simulink model "case3"  (R2024b)
settings: Solver=FixedStepAuto  StartTime=0  StopTime=1  FixedStep=1e-7  RelTol=1e-3
values from neighbouring files (symbols this model uses):
  SG_D_1_D = 0.01056    [IEEE9_case_parameters.m]    (also in case1_parameters.m; case2_parameters.m; case3_parameters.m; case4_parameters.m)
  SG_D_1_EnableSaturation = 0    [IEEE9_case_parameters.m]    (also in case1_parameters.m; case2_parameters.m; case3_parameters.m; case4_parameters.m)
  SG_D_1_f0 = 60    [IEEE9_case_parameters.m]    (also in case1_parameters.m; case2_parameters.m; case3_parameters.m; case4_parameters.m)
  SG_D_1_H = 7.5    [IEEE9_case_parameters.m]    (also in case1_parameters.m; case2_parameters.m; case3_parameters.m; case4_parameters.m)
  SG_D_1_K_A = 20    [IEEE9_case_parameters.m]    (also in case1_parameters.m; case2_parameters.m; case3_parameters.m; case4_parameters.m)
  SG_D_1_K_E = 1.000000e+1    (= 10)    [IEEE9_case_parameters.m]    (also in case1_parameters.m; case2_parameters.m; case3_parameters.m; case4_parameters.m)
  SG_D_1_K_F = 2.363    [IEEE9_case_parameters.m]    (also in case1_parameters.m; case2_parameters.m; case3_parameters.m; case4_parameters.m)
  SG_D_1_K_s = 0.5    [IEEE9_case_parameters.m]    (also in case1_parameters.m = 5; case2_parameters.m = 5; case3_parameters.m = 5; case4_parameters.m = 5)
  SG_D_1_R_a = 0.001088    [IEEE9_case_parameters.m]    (also in case1_parameters.m; case2_parameters.m; case3_parameters.m; case4_parameters.m)
  SG_D_1_S_A = 1    [IEEE9_case_parameters.m]    (also in case1_parameters.m; case2_parameters.m; case3_parameters.m; case4_parameters.m)
  SG_D_1_S_B = 0.103    [IEEE9_case_parameters.m]    (also in case1_parameters.m; case2_parameters.m; case3_parameters.m; case4_parameters.m)
  SG_D_1_S_N = 10.659857    [IEEE9_case_parameters.m]    (also in case1_parameters.m; case2_parameters.m; case3_parameters.m; case4_parameters.m)
  SG_D_1_SpeedPara = 200    [IEEE9_case_parameters.m]    (also in case1_parameters.m; case2_parameters.m; case3_parameters.m; case4_parameters.m)
  SG_D_1_T_0 = 0.720173    [IEEE9_case_parameters.m]    (also in case1_parameters.m = 0.755522; case2_parameters.m = 0.808931; case3_parameters.m = 0.869402; case4_parameters.m = 0.729316)
  SG_D_1_T_1 = 0.3    [IEEE9_case_parameters.m]    (also in case1_parameters.m; case2_parameters.m; case3_parameters.m; case4_parameters.m)
  SG_D_1_T_2 = 0.05    [IEEE9_case_parameters.m]    (also in case1_parameters.m; case2_parameters.m; case3_parameters.m; case4_parameters.m)
  SG_D_1_T_3 = 0.02    [IEEE9_case_parameters.m]    (also in case1_parameters.m; case2_parameters.m; case3_parameters.m; case4_parameters.m)
  SG_D_1_T_4 = 0.005    [IEEE9_case_parameters.m]    (also in case1_parameters.m; case2_parameters.m; case3_parameters.m; case4_parameters.m)
  SG_D_1_T_A = 0.02    [IEEE9_case_parameters.m]    (also in case1_parameters.m; case2_parameters.m; case3_parameters.m; case4_parameters.m)
  SG_D_1_T_dd = 8.000000e+0    (= 8)    [IEEE9_case_parameters.m]    (also in case1_parameters.m; case2_parameters.m; case3_parameters.m; case4_parameters.m)
  SG_D_1_T_ddd = 0.04    [IEEE9_case_parameters.m]    (also in case1_parameters.m; case2_parameters.m; case3_parameters.m; case4_parameters.m)
  SG_D_1_T_E = 0.314    [IEEE9_case_parameters.m]    (also in case1_parameters.m; case2_parameters.m; case3_parameters.m; case4_parameters.m)
  SG_D_1_T_F = 0.35    [IEEE9_case_parameters.m]    (also in case1_parameters.m; case2_parameters.m; case3_parameters.m; case4_parameters.m)
  SG_D_1_T_qd = 0.8    [IEEE9_case_parameters.m]    (also in case1_parameters.m; case2_parameters.m; case3_parameters.m; case4_parameters.m)
  SG_D_1_T_qdd = 0.02    [IEEE9_case_parameters.m]    (also in case1_parameters.m; case2_parameters.m; case3_parameters.m; case4_parameters.m)
  SG_D_1_T_speed = 0.1    [IEEE9_case_parameters.m]    (also in case1_parameters.m = 200; case2_parameters.m = 200; case3_parameters.m = 200; case4_parameters.m = 200)
  SG_D_1_T_w = 0.5    [IEEE9_case_parameters.m]    (also in case1_parameters.m; case2_parameters.m; case3_parameters.m; case4_parameters.m)
  SG_D_1_V_ref = 1.990276    [IEEE9_case_parameters.m]    (also in case1_parameters.m = 2.042296; case2_parameters.m = 2.051388; case3_parameters.m = 2.089584; case4_parameters.m = 2.01845)
  SG_D_1_w_ref = 376.991118    [IEEE9_case_parameters.m]    (also in case1_parameters.m; case2_parameters.m; case3_parameters.m; case4_parameters.m)
  SG_D_1_wb = 6.000000e+1    (= 60)    [IEEE9_case_parameters.m]    (also in case1_parameters.m; case2_parameters.m; case3_parameters.m; case4_parameters.m)
  SG_D_1_x_d = 1.9    [IEEE9_case_parameters.m]    (also in case1_parameters.m; case2_parameters.m; case3_parameters.m; case4_parameters.m)
  SG_D_1_x_dd = 0.302    [IEEE9_case_parameters.m]    (also in case1_parameters.m; case2_parameters.m; case3_parameters.m; case4_parameters.m)
  SG_D_1_x_ddd = 0.204    [IEEE9_case_parameters.m]    (also in case1_parameters.m; case2_parameters.m; case3_parameters.m; case4_parameters.m)
  SG_D_1_x_l = 0.05    [IEEE9_case_parameters.m]    (also in case1_parameters.m; case2_parameters.m; case3_parameters.m; case4_parameters.m)
  SG_D_1_x_q = 1.3    [IEEE9_case_parameters.m]    (also in case1_parameters.m; case2_parameters.m; case3_parameters.m; case4_parameters.m)
  SG_D_1_x_qd = 0.5    [IEEE9_case_parameters.m]    (also in case1_parameters.m; case2_parameters.m; case3_parameters.m; case4_parameters.m)
  SG_D_1_x_qdd = 0.3    [IEEE9_case_parameters.m]    (also in case1_parameters.m; case2_parameters.m; case3_parameters.m; case4_parameters.m)
  SG_D_2_D = 0.02    [IEEE9_case_parameters.m]    (also in case1_parameters.m; case2_parameters.m; case3_parameters.m; case4_parameters.m)
  SG_D_2_EnableSaturation = 0    [IEEE9_case_parameters.m]    (also in case1_parameters.m; case2_parameters.m; case3_parameters.m; case4_parameters.m)
  SG_D_2_f0 = 60    [IEEE9_case_parameters.m]    (also in case1_parameters.m; case2_parameters.m; case3_parameters.m; case4_parameters.m)
  SG_D_2_H = 8.000000e+0    (= 8)    [IEEE9_case_parameters.m]    (also in case1_parameters.m; case2_parameters.m; case3_parameters.m; case4_parameters.m)
  SG_D_2_K_A = 20    [IEEE9_case_parameters.m]    (also in case1_parameters.m; case2_parameters.m; case3_parameters.m; case4_parameters.m)
  SG_D_2_K_E = 1.000000e+1    (= 10)    [IEEE9_case_parameters.m]    (also in case1_parameters.m; case2_parameters.m; case3_parameters.m; case4_parameters.m)
  SG_D_2_K_F = 2.363    [IEEE9_case_parameters.m]    (also in case1_parameters.m; case2_parameters.m; case3_parameters.m; case4_parameters.m)
  SG_D_2_K_s = 0.5    [IEEE9_case_parameters.m]    (also in case1_parameters.m = 4; case2_parameters.m = 4; case3_parameters.m = 4; case4_parameters.m = 4)
  SG_D_2_R_a = 0.001088    [IEEE9_case_parameters.m]    (also in case1_parameters.m; case2_parameters.m; case3_parameters.m; case4_parameters.m)
  SG_D_2_S_A = 1    [IEEE9_case_parameters.m]    (also in case1_parameters.m; case2_parameters.m; case3_parameters.m; case4_parameters.m)
  SG_D_2_S_B = 0.103    [IEEE9_case_parameters.m]    (also in case1_parameters.m; case2_parameters.m; case3_parameters.m; case4_parameters.m)
  SG_D_2_S_N = 10.659857    [IEEE9_case_parameters.m]    (also in case1_parameters.m; case2_parameters.m; case3_parameters.m; case4_parameters.m)
  SG_D_2_SpeedPara = 200    [IEEE9_case_parameters.m]    (also in case1_parameters.m; case2_parameters.m; case3_parameters.m; case4_parameters.m)
  SG_D_2_T_0 = 1.632913    [IEEE9_case_parameters.m]    (also in case1_parameters.m = 1.632925; case2_parameters.m = 1.632915; case3_parameters.m = 1.632914; case4_parameters.m = 1.632927)
  SG_D_2_T_1 = 0.2    [IEEE9_case_parameters.m]    (also in case1_parameters.m; case2_parameters.m; case3_parameters.m; case4_parameters.m)
  SG_D_2_T_2 = 0.05    [IEEE9_case_parameters.m]    (also in case1_parameters.m; case2_parameters.m; case3_parameters.m; case4_parameters.m)
  SG_D_2_T_3 = 0.02    [IEEE9_case_parameters.m]    (also in case1_parameters.m; case2_parameters.m; case3_parameters.m; case4_parameters.m)
  SG_D_2_T_4 = 0.005    [IEEE9_case_parameters.m]    (also in case1_parameters.m; case2_parameters.m; case3_parameters.m; case4_parameters.m)
  SG_D_2_T_A = 0.02    [IEEE9_case_parameters.m]    (also in case1_parameters.m; case2_parameters.m; case3_parameters.m; case4_parameters.m)
  SG_D_2_T_dd = 7.9    [IEEE9_case_parameters.m]    (also in case1_parameters.m; case2_parameters.m; case3_parameters.m; case4_parameters.m)
  SG_D_2_T_ddd = 0.04    [IEEE9_case_parameters.m]    (also in case1_parameters.m; case2_parameters.m; case3_parameters.m; case4_parameters.m)
  SG_D_2_T_E = 0.314    [IEEE9_case_parameters.m]    (also in case1_parameters.m; case2_parameters.m; case3_parameters.m; case4_parameters.m)
  SG_D_2_T_F = 0.35    [IEEE9_case_parameters.m]    (also in case1_parameters.m; case2_parameters.m; case3_parameters.m; case4_parameters.m)
  SG_D_2_T_qd = 0.8    [IEEE9_case_parameters.m]    (also in case1_parameters.m; case2_parameters.m; case3_parameters.m; case4_parameters.m)
  SG_D_2_T_qdd = 0.015    [IEEE9_case_parameters.m]    (also in case1_parameters.m; case2_parameters.m; case3_parameters.m; case4_parameters.m)
  SG_D_2_T_speed = 0.1    [IEEE9_case_parameters.m]    (also in case1_parameters.m = 150; case2_parameters.m = 150; case3_parameters.m = 150; case4_parameters.m = 150)
  SG_D_2_T_w = 0.35    [IEEE9_case_parameters.m]    (also in case1_parameters.m; case2_parameters.m; case3_parameters.m; case4_parameters.m)
  SG_D_2_V_ref = 2.58547    [IEEE9_case_parameters.m]    (also in case1_parameters.m = 2.597896; case2_parameters.m = 2.587136; case3_parameters.m = 2.586042; case4_parameters.m = 2.599679)
  SG_D_2_w_ref = 376.991118    [IEEE9_case_parameters.m]    (also in case1_parameters.m; case2_parameters.m; case3_parameters.m; case4_parameters.m)
  SG_D_2_wb = 6.000000e+1    (= 60)    [IEEE9_case_parameters.m]    (also in case1_parameters.m; case2_parameters.m; case3_parameters.m; case4_parameters.m)
  SG_D_2_x_d = 1.8    [IEEE9_case_parameters.m]    (also in case1_parameters.m; case2_parameters.m; case3_parameters.m; case4_parameters.m)
  SG_D_2_x_dd = 0.302    [IEEE9_case_parameters.m]    (also in case1_parameters.m; case2_parameters.m; case3_parameters.m; case4_parameters.m)
  SG_D_2_x_ddd = 0.204    [IEEE9_case_parameters.m]    (also in case1_parameters.m; case2_parameters.m; case3_parameters.m; case4_parameters.m)
  SG_D_2_x_l = 0.05    [IEEE9_case_parameters.m]    (also in case1_parameters.m; case2_parameters.m; case3_parameters.m; case4_parameters.m)
  SG_D_2_x_q = 1.25    [IEEE9_case_parameters.m]    (also in case1_parameters.m; case2_parameters.m; case3_parameters.m; case4_parameters.m)
  SG_D_2_x_qd = 0.5    [IEEE9_case_parameters.m]    (also in case1_parameters.m; case2_parameters.m; case3_parameters.m; case4_parameters.m)
  SG_D_2_x_qdd = 0.3    [IEEE9_case_parameters.m]    (also in case1_parameters.m; case2_parameters.m; case3_parameters.m; case4_parameters.m)
  SG_D_3_D = 0.02    [IEEE9_case_parameters.m]    (also in case1_parameters.m; case2_parameters.m; case3_parameters.m; case4_parameters.m)
  SG_D_3_EnableSaturation = 0    [IEEE9_case_parameters.m]    (also in case1_parameters.m; case2_parameters.m; case3_parameters.m; case4_parameters.m)
  SG_D_3_f0 = 60    [IEEE9_case_parameters.m]    (also in case1_parameters.m; case2_parameters.m; case3_parameters.m; case4_parameters.m)
  SG_D_3_H = 7.7    [IEEE9_case_parameters.m]    (also in case1_parameters.m; case2_parameters.m; case3_parameters.m; case4_parameters.m)
  SG_D_3_K_A = 20    [IEEE9_case_parameters.m]    (also in case1_parameters.m; case2_parameters.m; case3_parameters.m; case4_parameters.m)
  SG_D_3_K_E = 1.000000e+1    (= 10)    [IEEE9_case_parameters.m]    (also in case1_parameters.m; case2_parameters.m; case3_parameters.m; case4_parameters.m)
  SG_D_3_K_F = 2.363    [IEEE9_case_parameters.m]    (also in case1_parameters.m; case2_parameters.m; case3_parameters.m; case4_parameters.m)
  SG_D_3_K_s = 0.2    [IEEE9_case_parameters.m]    (also in case1_parameters.m = 2; case2_parameters.m = 2; case3_parameters.m = 2; case4_parameters.m = 2)
  SG_D_3_R_a = 0.001088    [IEEE9_case_parameters.m]    (also in case1_parameters.m; case2_parameters.m; case3_parameters.m; case4_parameters.m)
  SG_D_3_S_A = 1    [IEEE9_case_parameters.m]    (also in case1_parameters.m; case2_parameters.m; case3_parameters.m; case4_parameters.m)
  SG_D_3_S_B = 0.103    [IEEE9_case_parameters.m]    (also in case1_parameters.m; case2_parameters.m; case3_parameters.m; case4_parameters.m)
  SG_D_3_S_N = 10.659857    [IEEE9_case_parameters.m]    (also in case1_parameters.m; case2_parameters.m; case3_parameters.m; case4_parameters.m)
  SG_D_3_SpeedPara = 200    [IEEE9_case_parameters.m]    (also in case1_parameters.m; case2_parameters.m; case3_parameters.m; case4_parameters.m)
  SG_D_3_T_0 = 0.850788    [IEEE9_case_parameters.m]    (also in case1_parameters.m = 0.850786; case2_parameters.m = 0.850787; case3_parameters.m; case4_parameters.m = 0.850786)
  SG_D_3_T_1 = 0.2    [IEEE9_case_parameters.m]    (also in case1_parameters.m; case2_parameters.m; case3_parameters.m; case4_parameters.m)
  SG_D_3_T_2 = 0.05    [IEEE9_case_parameters.m]    (also in case1_parameters.m; case2_parameters.m; case3_parameters.m; case4_parameters.m)
  SG_D_3_T_3 = 0.02    [IEEE9_case_parameters.m]    (also in case1_parameters.m; case2_parameters.m; case3_parameters.m; case4_parameters.m)
  SG_D_3_T_4 = 0.005    [IEEE9_case_parameters.m]    (also in case1_parameters.m; case2_parameters.m; case3_parameters.m; case4_parameters.m)
  SG_D_3_T_A = 0.02    [IEEE9_case_parameters.m]    (also in case1_parameters.m; case2_parameters.m; case3_parameters.m; case4_parameters.m)
  SG_D_3_T_dd = 8.1    [IEEE9_case_parameters.m]    (also in case1_parameters.m; case2_parameters.m; case3_parameters.m; case4_parameters.m)
  SG_D_3_T_ddd = 0.04    [IEEE9_case_parameters.m]    (also in case1_parameters.m; case2_parameters.m; case3_parameters.m; case4_parameters.m)
  SG_D_3_T_E = 0.314    [IEEE9_case_parameters.m]    (also in case1_parameters.m; case2_parameters.m; case3_parameters.m; case4_parameters.m)
  SG_D_3_T_F = 0.35    [IEEE9_case_parameters.m]    (also in case1_parameters.m; case2_parameters.m; case3_parameters.m; case4_parameters.m)
  SG_D_3_T_qd = 0.8    [IEEE9_case_parameters.m]    (also in case1_parameters.m; case2_parameters.m; case3_parameters.m; case4_parameters.m)
  SG_D_3_T_qdd = 0.015    [IEEE9_case_parameters.m]    (also in case1_parameters.m; case2_parameters.m; case3_parameters.m; case4_parameters.m)
  SG_D_3_T_speed = 0.1    [IEEE9_case_parameters.m]    (also in case1_parameters.m = 180; case2_parameters.m = 180; case3_parameters.m = 180; case4_parameters.m = 180)
  SG_D_3_T_w = 0.4    [IEEE9_case_parameters.m]    (also in case1_parameters.m; case2_parameters.m; case3_parameters.m; case4_parameters.m)
  SG_D_3_V_ref = 1.892727    [IEEE9_case_parameters.m]    (also in case1_parameters.m = 1.906439; case2_parameters.m = 1.895535; case3_parameters.m = 1.892105; case4_parameters.m = 1.906598)
  SG_D_3_w_ref = 376.991118    [IEEE9_case_parameters.m]    (also in case1_parameters.m; case2_parameters.m; case3_parameters.m; case4_parameters.m)
  SG_D_3_wb = 6.000000e+1    (= 60)    [IEEE9_case_parameters.m]    (also in case1_parameters.m; case2_parameters.m; case3_parameters.m; case4_parameters.m)
  SG_D_3_x_d = 1.85    [IEEE9_case_parameters.m]    (also in case1_parameters.m; case2_parameters.m; case3_parameters.m; case4_parameters.m)
  SG_D_3_x_dd = 0.302    [IEEE9_case_parameters.m]    (also in case1_parameters.m; case2_parameters.m; case3_parameters.m; case4_parameters.m)
  SG_D_3_x_ddd = 0.204    [IEEE9_case_parameters.m]    (also in case1_parameters.m; case2_parameters.m; case3_parameters.m; case4_parameters.m)
  SG_D_3_x_l = 0.05    [IEEE9_case_parameters.m]    (also in case1_parameters.m; case2_parameters.m; case3_parameters.m; case4_parameters.m)
  SG_D_3_x_q = 1.2    [IEEE9_case_parameters.m]    (also in case1_parameters.m; case2_parameters.m; case3_parameters.m; case4_parameters.m)
  SG_D_3_x_qd = 0.5    [IEEE9_case_parameters.m]    (also in case1_parameters.m; case2_parameters.m; case3_parameters.m; case4_parameters.m)
  SG_D_3_x_qdd = 0.3    [IEEE9_case_parameters.m]    (also in case1_parameters.m; case2_parameters.m; case3_parameters.m; case4_parameters.m)
(part 8 of 12)

== system case3/SG_D_2/d_psi_d_SG_D_2_block ==
  note: d_psi_d_SG_D_2 in case3
      | $2\,\pi \,f_{0}\,\left(v_{d,\mathrm{SG},D,2}\,\sin\left(\theta _{\mathrm{SG},D,2}\right)-v_{q,\mathrm{SG},D,2}\,\cos\left(\theta _{\mathrm{SG},D,2}\right)+\frac{R_{a}\,\left(\frac{\psi _{\mathrm{1d},\mathrm{SG},D,2}\,\left(x_{\mathrm{dd}}-x_{\mathrm{ddd}}\right)}{x_{\mathrm{dd}}-x_{l}}-\psi _{d,\mathrm{SG},D,2}+\frac{\psi _{\mathrm{fd},\mathrm{SG},D,2}\,\left(x_{\mathrm{ddd}}-x_{l}\right)}{x_{\mathrm{dd}}-x_{l}}\right)}{x_{\mathrm{ddd}}}+\frac{\psi _{q,\mathrm{SG},D,2}\,w_{\mathrm{SG},D,2}}{2\,f_{0}\,\pi }\right)$
      | Automatically generated on 2025-10-31 18:59:51 .
  State_psi_1d_SG_D_2_d85f5 : Inport
  State_psi_d_SG_D_2_2712a : Inport  Port=2
  State_psi_fd_SG_D_2_3f7c9 : Inport  Port=3
  Input_v_d_SG_D_2_8a747 : Inport  Port=4
  State_theta_SG_D_2_fc879 : Inport  Port=5
  Input_v_q_SG_D_2_bd396 : Inport  Port=6
  State_theta_SG_D_2_1886b : Inport  Port=7
  State_psi_q_SG_D_2_f5763 : Inport  Port=8
  State_w_SG_D_2_5f49e : Inport  Port=9
  Add_4c6a2 : Sum
  Add_a24d9 : Sum
  Constant_-1_feb9b : Constant  Value=-1
  Constant_-2.0_5ab6a : Constant  Value=-2.0
  Constant_2.0_914c1 : Constant  Value=2.0
  Constant_R_a_7ff2e : Constant  Value=R_a
  Constant_f0_1428f : Constant  Value=f0
  Constant_f0_1bd3e : Constant  Value=f0
  Constant_pi_05147 : Constant  Value=pi
  Constant_pi_d2189 : Constant  Value=pi
  Constant_x_dd_3b685 : Constant  Value=x_dd
  Constant_x_dd_d1044 : Constant  Value=x_dd
  Constant_x_dd_fa650 : Constant  Value=x_dd
  Constant_x_ddd_117c4 : Constant  Value=x_ddd
  Constant_x_ddd_cc768 : Constant  Value=x_ddd
  Constant_x_ddd_feb60 : Constant  Value=x_ddd
  Constant_x_l_14631 : Constant  Value=x_l
  Constant_x_l_2aec7 : Constant  Value=x_l
  Constant_x_l_a18c8 : Constant  Value=x_l
  Divide_3d9c5 : Product  Inputs=*/
  Divide_6089c : Product  Inputs=*/
  Divide_65062 : Product  Inputs=*/
  Divide_be36f : Product  Inputs=*/
  MathFunc_cos_04d6f : Trigonometry  Operator=cos
  MathFunc_sin_14dfb : Trigonometry
  Product_01511 : Product
  Product_10db0 : Product
  Product_37ec0 : Product
  Product_3b24f : Product
  Product_8fc40 : Product
  Product_9439a : Product
  Product_a26ec : Product
  Product_ac62c : Product
  Product_c5a2d : Product
  Product_ce558 : Product
  Product_f0562 : Product
  Product_fc08e : Product
  Subtract_b11ba : Sum  Inputs=+-
  Subtract_b54f5 : Sum  Inputs=+-
  Subtract_c385c : Sum  Inputs=+-
  Subtract_c4546 : Sum  Inputs=+-
  Subtract_cb197 : Sum  Inputs=+-
  Subtract_e677e : Sum  Inputs=+-
  Subtract_ec460 : Sum  Inputs=+-
  Blockout_d_psi_d_SG_D_2_7b72e : Outport
  wires:
  MathFunc_sin_14dfb/1 -> Product_ce558/2
  Constant_x_dd_fa650/1 -> Subtract_c4546/1
  Constant_-1_feb9b/1 -> Product_01511/1
  Constant_x_l_2aec7/1 -> Subtract_c4546/2
  State_psi_1d_SG_D_2_d85f5/1 -> Product_01511/2
  Constant_f0_1428f/1 -> Product_c5a2d/2
  Constant_2.0_914c1/1 -> Product_fc08e/1
  Constant_x_l_a18c8/1 -> Subtract_e677e/2
  Constant_x_dd_3b685/1 -> Subtract_b54f5/1
  Product_f0562/1 -> Blockout_d_psi_d_SG_D_2_7b72e/1
  Constant_pi_d2189/1 -> Product_fc08e/2
  Constant_x_ddd_cc768/1 -> Subtract_b54f5/2
  Subtract_c385c/1 -> Product_f0562/2
  Product_01511/1 -> Product_8fc40/1
  Product_fc08e/1 -> Product_a26ec/1
  Subtract_b54f5/1 -> Product_8fc40/2
  Divide_3d9c5/1 -> Subtract_c385c/2
  Constant_x_ddd_117c4/1 -> Subtract_cb197/1
  Constant_x_l_14631/1 -> Subtract_cb197/2
  Product_8fc40/1 -> Divide_65062/1
  Subtract_ec460/1 -> Add_a24d9/1
  Subtract_c4546/1 -> Divide_65062/2
  State_psi_fd_SG_D_2_3f7c9/1 -> Product_ac62c/1
  Subtract_cb197/1 -> Product_ac62c/2
  Constant_x_dd_d1044/1 -> Subtract_e677e/1
  Divide_65062/1 -> Add_4c6a2/1
  State_psi_d_SG_D_2_2712a/1 -> Add_4c6a2/2
  Product_ac62c/1 -> Divide_6089c/1
  Subtract_e677e/1 -> Divide_6089c/2
  Add_4c6a2/1 -> Subtract_b11ba/1
  Divide_6089c/1 -> Subtract_b11ba/2
  Constant_R_a_7ff2e/1 -> Product_10db0/1
  Subtract_b11ba/1 -> Product_10db0/2
  Divide_be36f/1 -> Subtract_ec460/1
  State_theta_SG_D_2_fc879/1 -> MathFunc_sin_14dfb/1
  Product_10db0/1 -> Divide_be36f/1
  Constant_-2.0_5ab6a/1 -> Product_37ec0/1
  Input_v_d_SG_D_2_8a747/1 -> Product_ce558/1
  Constant_x_ddd_feb60/1 -> Divide_be36f/2
  State_theta_SG_D_2_1886b/1 -> MathFunc_cos_04d6f/1
  Product_c5a2d/1 -> Product_f0562/1
  Product_ce558/1 -> Subtract_ec460/2
  Product_37ec0/1 -> Product_c5a2d/1
  Input_v_q_SG_D_2_bd396/1 -> Product_9439a/1
  MathFunc_cos_04d6f/1 -> Product_9439a/2
  State_psi_q_SG_D_2_f5763/1 -> Product_3b24f/1
  State_w_SG_D_2_5f49e/1 -> Product_3b24f/2
  Constant_f0_1bd3e/1 -> Product_a26ec/2
  Constant_pi_05147/1 -> Product_37ec0/2
  Product_9439a/1 -> Add_a24d9/2
  Product_3b24f/1 -> Divide_3d9c5/1
  Product_a26ec/1 -> Divide_3d9c5/2
  Add_a24d9/1 -> Subtract_c385c/1

== system case3/SG_D_2/d_psi_fd_SG_D_2_block ==
  note: d_psi_fd_SG_D_2 in case3
      | $-\frac{\psi _{\mathrm{fd},\mathrm{SG},D,2}-E_{\mathrm{fd},\mathrm{SG},D,2}+\left(x_{d}-x_{\mathrm{dd}}\right)\,\left(\frac{\frac{\psi _{\mathrm{1d},\mathrm{SG},D,2}\,\left(x_{\mathrm{dd}}-x_{\mathrm{ddd}}\right)}{x_{\mathrm{dd}}-x_{l}}-\psi _{d,\mathrm{SG},D,2}+\frac{\psi _{\mathrm{fd},\mathrm{SG},D,2}\,\left(x_{\mathrm{ddd}}-x_{l}\right)}{x_{\mathrm{dd}}-x_{l}}}{x_{\mathrm{ddd}}}-\frac{\left(x_{\mathrm{dd}}-x_{\mathrm{ddd}}\right)\,\left(\psi _{\mathrm{1d},\mathrm{SG},D,2}-\psi _{\mathrm{fd},\mathrm{SG},D,2}+\frac{\left(x_{\mathrm{dd}}-x_{l}\right)\,\left(\frac{\psi _{\mathrm{1d},\mathrm{SG},D,2}\,\left(x_{\mathrm{dd}}-x_{\mathrm{ddd}}\right)}{x_{\mathrm{dd}}-x_{l}}-\psi _{d,\mathrm{SG},D,2}+\frac{\psi _{\mathrm{fd},\mathrm{SG},D,2}\,\left(x_{\mathrm{ddd}}-x_{l}\right)}{x_{\mathrm{dd}}-x_{l}}\right)}{x_{\mathrm{ddd}}}\right)}{{\left(x_{\mathrm{dd}}-x_{l}\right)}^2}\right)}{T_{\mathrm{dd}}}$
      | Automatically generated on 2025-10-31 19:00:00 .
  State_E_fd_SG_D_2_53335 : Inport
  State_psi_fd_SG_D_2_f7b95 : Inport  Port=2
  State_psi_1d_SG_D_2_7e7b9 : Inport  Port=3
  State_psi_fd_SG_D_2_eba15 : Inport  Port=4
  State_psi_1d_SG_D_2_899e2 : Inport  Port=5
  State_psi_d_SG_D_2_990fd : Inport  Port=6
  State_psi_fd_SG_D_2_f0ae5 : Inport  Port=7
  State_psi_1d_SG_D_2_9ae7e : Inport  Port=8
  State_psi_d_SG_D_2_3b4a4 : Inport  Port=9
  State_psi_fd_SG_D_2_a82ed : Inport  Port=10
  Add_568a9 : Sum
  Add_ca5e3 : Sum
  Constant_-1_28e45 : Constant  Value=-1
  Constant_-1_4ebc6 : Constant  Value=-1
  Constant_-1_db2ff : Constant  Value=-1
  Constant_2.0_70520 : Constant  Value=2.0
  Constant_T_dd_0bec4 : Constant  Value=T_dd
  Constant_x_d_9e043 : Constant  Value=x_d
  Constant_x_dd_01096 : Constant  Value=x_dd
  Constant_x_dd_081b1 : Constant  Value=x_dd
  Constant_x_dd_35849 : Constant  Value=x_dd
  Constant_x_dd_52851 : Constant  Value=x_dd
  Constant_x_dd_77a63 : Constant  Value=x_dd
  Constant_x_dd_94409 : Constant  Value=x_dd
  Constant_x_dd_a56a6 : Constant  Value=x_dd
  Constant_x_dd_bc6c4 : Constant  Value=x_dd
  Constant_x_dd_d29d6 : Constant  Value=x_dd
  Constant_x_dd_e0e8e : Constant  Value=x_dd
  Constant_x_ddd_6e182 : Constant  Value=x_ddd
  Constant_x_ddd_92e40 : Constant  Value=x_ddd
  Constant_x_ddd_92f17 : Constant  Value=x_ddd
  Constant_x_ddd_b3ae3 : Constant  Value=x_ddd
  Constant_x_ddd_ce1fb : Constant  Value=x_ddd
  Constant_x_ddd_d5210 : Constant  Value=x_ddd
  Constant_x_ddd_f595b : Constant  Value=x_ddd
  Constant_x_l_0c30d : Constant  Value=x_l
  Constant_x_l_1713e : Constant  Value=x_l
  Constant_x_l_86642 : Constant  Value=x_l
  Constant_x_l_8c7a2 : Constant  Value=x_l
  Constant_x_l_b0284 : Constant  Value=x_l
  Constant_x_l_b12d0 : Constant  Value=x_l
  Constant_x_l_d242d : Constant  Value=x_l
  Constant_x_l_f1e83 : Constant  Value=x_l
  Divide_1aca2 : Product  Inputs=*/
  Divide_8872e : Product  Inputs=*/
  Divide_93fdb : Product  Inputs=*/
  Divide_9bc65 : Product  Inputs=*/
  Divide_ca1d6 : Product  Inputs=*/
  Divide_d24c1 : Product  Inputs=*/
  Divide_d9c57 : Product  Inputs=*/
  Divide_e4f44 : Product  Inputs=*/
  Power_5f0d6 : Math  Operator=pow
  Product_2ea05 : Product
  Product_3add5 : Product
  Product_6f388 : Product
  Product_7e1ca : Product
  Product_97bca : Product
  Product_c22ea : Product
  Product_da1a5 : Product
  Product_e6966 : Product
  Product_f1bcc : Product
  Product_f509c : Product
  Subtract_1bae5 : Sum  Inputs=+-
  Subtract_219cd : Sum  Inputs=+-
  Subtract_21c97 : Sum  Inputs=+-
  Subtract_22d3d : Sum  Inputs=+-
  Subtract_232fa : Sum  Inputs=+-
  Subtract_2af62 : Sum  Inputs=+-
  Subtract_2bfb5 : Sum  Inputs=+-
  Subtract_34813 : Sum  Inputs=+-
  Subtract_3a4c2 : Sum  Inputs=+-
  Subtract_3b31a : Sum  Inputs=+-
  Subtract_3fdcd : Sum  Inputs=+-
  Subtract_5c31b : Sum  Inputs=+-
  Subtract_673a5 : Sum  Inputs=+-
  Subtract_98e0f : Sum  Inputs=+-
  Subtract_a52d6 : Sum  Inputs=+-
  Subtract_c28ba : Sum  Inputs=+-
  Subtract_cdf6b : Sum  Inputs=+-
  Subtract_ceaa9 : Sum  Inputs=+-
  Subtract_fcd4f : Sum  Inputs=+-
  Blockout_d_psi_fd_SG_D_2_efff3 : Outport
  wires:
  Constant_x_dd_52851/1 -> Subtract_a52d6/1
  Constant_-1_28e45/1 -> Product_f509c/1
  Constant_x_l_b0284/1 -> Subtract_c28ba/2
  Divide_1aca2/1 -> Add_ca5e3/1
  Subtract_2bfb5/1 -> Product_da1a5/2
  Constant_x_l_b12d0/1 -> Subtract_a52d6/2
  Product_da1a5/1 -> Divide_d24c1/1
  State_psi_1d_SG_D_2_899e2/1 -> Product_f509c/2
  Constant_x_dd_e0e8e/1 -> Subtract_3a4c2/1
  Product_c22ea/1 -> Divide_1aca2/1
  Constant_x_dd_a56a6/1 -> Subtract_34813/1
  Constant_x_ddd_92e40/1 -> Subtract_3a4c2/2
  Constant_x_dd_01096/1 -> Subtract_21c97/1
  Product_f509c/1 -> Product_97bca/1
  Subtract_3a4c2/1 -> Product_97bca/2
  State_psi_d_SG_D_2_3b4a4/1 -> Add_ca5e3/2
  Constant_x_ddd_6e182/1 -> Subtract_2bfb5/1
  Constant_x_l_8c7a2/1 -> Subtract_2bfb5/2
  Product_97bca/1 -> Divide_93fdb/1
  Subtract_a52d6/1 -> Divide_93fdb/2
  State_psi_fd_SG_D_2_f0ae5/1 -> Product_da1a5/1
  Subtract_cdf6b/1 -> Product_3add5/2
  Constant_x_dd_94409/1 -> Subtract_22d3d/1
  Constant_x_l_0c30d/1 -> Subtract_22d3d/2
  Product_2ea05/1 -> Product_3add5/1
  Divide_93fdb/1 -> Add_568a9/1
  State_psi_d_SG_D_2_990fd/1 -> Add_568a9/2
  Subtract_22d3d/1 -> Divide_d24c1/2
  Constant_x_dd_77a63/1 -> Subtract_c28ba/1
  Constant_x_ddd_b3ae3/1 -> Subtract_2af62/1
  Add_568a9/1 -> Subtract_fcd4f/1
  Divide_d24c1/1 -> Subtract_fcd4f/2
  Constant_-1_4ebc6/1 -> Product_e6966/1
  Product_6f388/1 -> Divide_8872e/1
  State_psi_1d_SG_D_2_9ae7e/1 -> Product_e6966/2
  Subtract_34813/1 -> Product_2ea05/2
  Constant_x_dd_35849/1 -> Subtract_1bae5/1
  Divide_8872e/1 -> Subtract_219cd/2
  Constant_-1_db2ff/1 -> Product_2ea05/1
  Constant_x_ddd_ce1fb/1 -> Subtract_1bae5/2
  Constant_x_ddd_f595b/1 -> Divide_e4f44/2
  Subtract_c28ba/1 -> Product_7e1ca/1
  Subtract_fcd4f/1 -> Product_7e1ca/2
  State_psi_fd_SG_D_2_eba15/1 -> Subtract_3fdcd/2
  Product_e6966/1 -> Product_c22ea/1
  Subtract_1bae5/1 -> Product_c22ea/2
  Constant_2.0_70520/1 -> Power_5f0d6/2
  State_psi_1d_SG_D_2_7e7b9/1 -> Subtract_3fdcd/1
  Constant_x_dd_bc6c4/1 -> Subtract_98e0f/1
  Subtract_2af62/1 -> Product_6f388/2
  Constant_x_l_d242d/1 -> Subtract_98e0f/2
  Constant_x_l_f1e83/1 -> Subtract_2af62/2
  Constant_x_ddd_92f17/1 -> Subtract_34813/2
  Subtract_21c97/1 -> Divide_8872e/2
  Product_7e1ca/1 -> Divide_e4f44/1
  Subtract_98e0f/1 -> Divide_1aca2/2
  State_psi_fd_SG_D_2_a82ed/1 -> Product_6f388/1
  Constant_x_l_1713e/1 -> Subtract_21c97/2
  Constant_x_dd_d29d6/1 -> Subtract_ceaa9/1
  Subtract_3fdcd/1 -> Subtract_cdf6b/1
  Divide_e4f44/1 -> Subtract_cdf6b/2
  Constant_x_l_86642/1 -> Subtract_ceaa9/2
  Subtract_ceaa9/1 -> Power_5f0d6/1
  Add_ca5e3/1 -> Subtract_219cd/1
  Product_3add5/1 -> Divide_9bc65/1
  Power_5f0d6/1 -> Divide_9bc65/2
  Subtract_219cd/1 -> Divide_d9c57/1
  Constant_x_ddd_d5210/1 -> Divide_d9c57/2
  Constant_x_d_9e043/1 -> Subtract_673a5/1
  Constant_x_dd_081b1/1 -> Subtract_673a5/2
  Divide_9bc65/1 -> Subtract_232fa/1
  Divide_d9c57/1 -> Subtract_232fa/2
  State_E_fd_SG_D_2_53335/1 -> Subtract_3b31a/1
  State_psi_fd_SG_D_2_f7b95/1 -> Subtract_3b31a/2
  Subtract_673a5/1 -> Product_f1bcc/1
  Subtract_232fa/1 -> Product_f1bcc/2
  Subtract_3b31a/1 -> Subtract_5c31b/1
  Product_f1bcc/1 -> Subtract_5c31b/2
  Subtract_5c31b/1 -> Divide_ca1d6/1
  Constant_T_dd_0bec4/1 -> Divide_ca1d6/2
  Divide_ca1d6/1 -> Blockout_d_psi_fd_SG_D_2_efff3/1

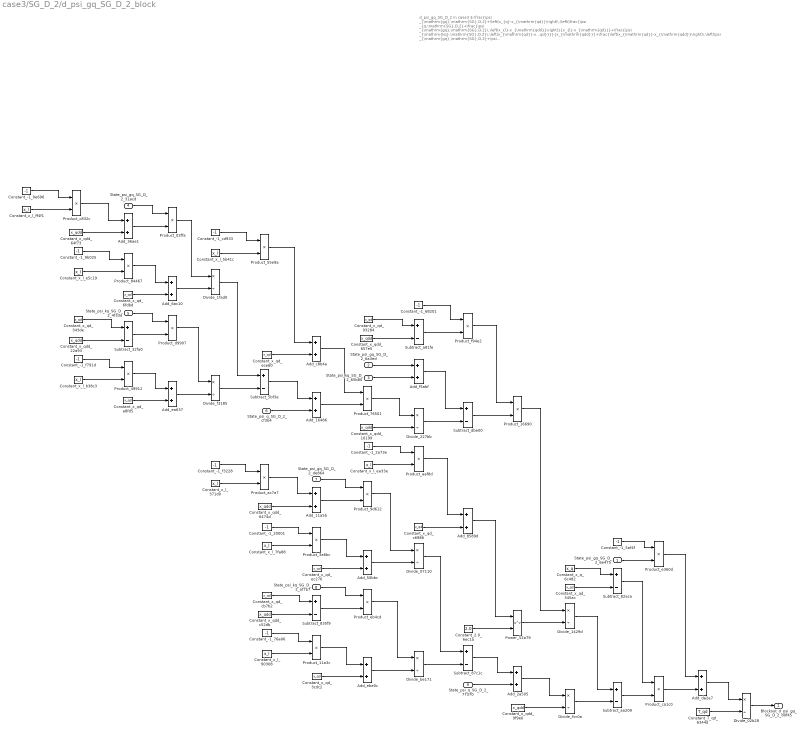
== system case3/SG_D_2/d_psi_gq_SG_D_2_block ==
  note: d_psi_gq_SG_D_2 in case3
      | $-\frac{\psi _{\mathrm{gq},\mathrm{SG},D,2}+\left(x_{q}-x_{\mathrm{qd}}\right)\,\left(\frac{\psi _{q,\mathrm{SG},D,2}+\frac{\psi _{\mathrm{gq},\mathrm{SG},D,2}\,\left(x_{l}-x_{\mathrm{qdd}}\right)}{x_{l}-x_{\mathrm{qd}}}+\frac{\psi _{\mathrm{kq},\mathrm{SG},D,2}\,\left(x_{\mathrm{qd}}-x_{\mathrm{qdd}}\right)}{x_{l}-x_{\mathrm{qd}}}}{x_{\mathrm{qdd}}}+\frac{\left(x_{\mathrm{qd}}-x_{\mathrm{qdd}}\right)\,\left(\psi _{\mathrm{gq},\mathrm{SG},D,2}+\psi _{\mathrm{kq},\mathrm{SG},D,2}+\frac{\left(x_{l}-x_{\mathrm{qd}}\right)\,\left(\psi _{q,\mathrm{SG},D,2}+\frac{\psi _{\mathrm{gq},\mathrm{SG},D,2}\,\left(x_{l}-x_{\mathrm{qdd}}\right)}{x_{l}-x_{\mathrm{qd}}}+\frac{\psi _{\mathrm{kq},\mathrm{SG},D,2}\,\left(x_{\mathrm{qd}}-x_{\mathrm{qdd}}\right)}{x_{l}-x_{\mathrm{qd}}}\right)}{x_{\mathrm{qdd}}}\right)}{{\left(x_{l}-x_{\mathrm{qd}}\right)}^2}\right)}{T_{\mathrm{qd}}}$
      | Automatically generated on 2025-10-31 19:00:09 .
  State_psi_gq_SG_D_2_6e475 : Inport
  State_psi_gq_SG_D_2_6a3ed : Inport  Port=2
  State_psi_kq_SG_D_2_65b80 : Inport  Port=3
  State_psi_gq_SG_D_2_31acd : Inport  Port=4
  State_psi_kq_SG_D_2_4f33d : Inport  Port=5
  State_psi_q_SG_D_2_cf3b4 : Inport  Port=6
  State_psi_gq_SG_D_2_de864 : Inport  Port=7
  State_psi_kq_SG_D_2_af7b7 : Inport  Port=8
  State_psi_q_SG_D_2_77370 : Inport  Port=9
  Add_11a5b : Sum
  Add_16486 : Sum
  Add_2a505 : Sum
  Add_36ae1 : Sum
  Add_50bbc : Sum
  Add_6ac10 : Sum
  Add_8589d : Sum
  Add_c8b4a : Sum
  Add_da2e7 : Sum
  Add_ea637 : Sum
  Add_ebe0c : Sum
  Add_f5abf : Sum
  Constant_-1_0e696 : Constant  Value=-1
  Constant_-1_20001 : Constant  Value=-1
  Constant_-1_2a73e : Constant  Value=-1
  Constant_-1_5af4f : Constant  Value=-1
  Constant_-1_68201 : Constant  Value=-1
  Constant_-1_76a06 : Constant  Value=-1
  Constant_-1_9b025 : Constant  Value=-1
  Constant_-1_cd933 : Constant  Value=-1
  Constant_-1_f3228 : Constant  Value=-1
  Constant_-1_f791d : Constant  Value=-1
  Constant_2.0_6ec1a : Constant  Value=2.0
  Constant_T_qd_6344d : Constant  Value=T_qd
  Constant_x_l_371d0 : Constant  Value=x_l
  Constant_x_l_5b41c : Constant  Value=x_l
  Constant_x_l_7fa88 : Constant  Value=x_l
  Constant_x_l_90308 : Constant  Value=x_l
  Constant_x_l_b38c3 : Constant  Value=x_l
  Constant_x_l_e5c19 : Constant  Value=x_l
  Constant_x_l_ea33e : Constant  Value=x_l
  Constant_x_l_ff4f1 : Constant  Value=x_l
  Constant_x_q_6c482 : Constant  Value=x_q
  Constant_x_qd_343de : Constant  Value=x_qd
  Constant_x_qd_345ac : Constant  Value=x_qd
  Constant_x_qd_3cdc2 : Constant  Value=x_qd
  Constant_x_qd_6fdbd : Constant  Value=x_qd
  Constant_x_qd_93284 : Constant  Value=x_qd
  Constant_x_qd_a8fd5 : Constant  Value=x_qd
  Constant_x_qd_c6986 : Constant  Value=x_qd
  Constant_x_qd_cb7b2 : Constant  Value=x_qd
  Constant_x_qd_ec276 : Constant  Value=x_qd
  Constant_x_qd_ece60 : Constant  Value=x_qd
  Constant_x_qdd_16199 : Constant  Value=x_qdd
  Constant_x_qdd_22a93 : Constant  Value=x_qdd
  Constant_x_qdd_6474d : Constant  Value=x_qdd
  Constant_x_qdd_64f73 : Constant  Value=x_qdd
  Constant_x_qdd_657e5 : Constant  Value=x_qdd
  Constant_x_qdd_9f9e6 : Constant  Value=x_qdd
  Constant_x_qdd_c52db : Constant  Value=x_qdd
  Divide_02b28 : Product  Inputs=*/
  Divide_07110 : Product  Inputs=*/
  Divide_1429d : Product  Inputs=*/
  Divide_1fad0 : Product  Inputs=*/
  Divide_227bb : Product  Inputs=*/
  Divide_be171 : Product  Inputs=*/
  Divide_f3185 : Product  Inputs=*/
  Divide_fcc0a : Product  Inputs=*/
  Power_52a79 : Math  Operator=pow
  Product_03ffa : Product
  Product_11a3c : Product
  Product_{16690,49912,76501,84467} (4 alike) : Product
  Product_3a6bc : Product
  Product_55e9a : Product
  Product_9d612 : Product
  Product_aaf8d : Product
  Product_ac7a7 : Product
  Product_c832c : Product
  Product_ca1c0 : Product
  Product_d9907 : Product
  Product_e360d : Product
  Product_eb4cd : Product
  Product_f94e2 : Product
  Subtract_32fa0 : Sum  Inputs=+-
  Subtract_5bf3e : Sum  Inputs=+-
  Subtract_82aca : Sum  Inputs=+-
  Subtract_835f9 : Sum  Inputs=+-
  Subtract_87c1c : Sum  Inputs=+-
  Subtract_a81fe : Sum  Inputs=+-
  Subtract_aa209 : Sum  Inputs=+-
  Subtract_dbe00 : Sum  Inputs=+-
  Blockout_d_psi_gq_SG_D_2_d0f45 : Outport
  wires:
  Constant_x_l_90308/1 -> Product_11a3c/2
  Constant_x_l_371d0/1 -> Product_ac7a7/2
  Constant_x_qd_343de/1 -> Subtract_32fa0/1
  Constant_x_l_ea33e/1 -> Product_aaf8d/2
  Constant_x_qdd_657e5/1 -> Subtract_a81fe/2
  Constant_-1_f791d/1 -> Product_49912/1
  Constant_-1_0e696/1 -> Product_c832c/1
  State_psi_gq_SG_D_2_6a3ed/1 -> Add_f5abf/1
  Constant_x_qdd_22a93/1 -> Subtract_32fa0/2
  Constant_x_qd_93284/1 -> Subtract_a81fe/1
  Constant_x_l_b38c3/1 -> Product_49912/2
  Constant_x_l_ff4f1/1 -> Product_c832c/2
  Product_49912/1 -> Add_ea637/1
  Product_c832c/1 -> Add_36ae1/1
  Constant_x_l_e5c19/1 -> Product_84467/2
  Constant_x_l_5b41c/1 -> Product_55e9a/2
  Constant_x_qd_a8fd5/1 -> Add_ea637/2
  Constant_x_qdd_64f73/1 -> Add_36ae1/2
  Constant_-1_9b025/1 -> Product_84467/1
  Constant_x_qd_3cdc2/1 -> Add_ebe0c/2
  Constant_x_qdd_6474d/1 -> Add_11a5b/2
  State_psi_gq_SG_D_2_31acd/1 -> Product_03ffa/1
  Add_ea637/1 -> Divide_f3185/2
  Add_36ae1/1 -> Product_03ffa/2
  Constant_x_qd_345ac/1 -> Subtract_82aca/2
  Product_84467/1 -> Add_6ac10/1
  Constant_x_qd_6fdbd/1 -> Add_6ac10/2
  State_psi_kq_SG_D_2_4f33d/1 -> Product_d9907/1
  Divide_1fad0/1 -> Subtract_5bf3e/1
  Subtract_32fa0/1 -> Product_d9907/2
  Product_03ffa/1 -> Divide_1fad0/1
  Add_6ac10/1 -> Divide_1fad0/2
  Add_16486/1 -> Product_76501/2
  Product_d9907/1 -> Divide_f3185/1
  Constant_-1_cd933/1 -> Product_55e9a/1
  Divide_f3185/1 -> Subtract_5bf3e/2
  Constant_-1_76a06/1 -> Product_11a3c/1
  Constant_-1_f3228/1 -> Product_ac7a7/1
  Product_55e9a/1 -> Add_c8b4a/1
  Constant_x_qdd_c52db/1 -> Subtract_835f9/2
  Constant_x_qd_ece60/1 -> Add_c8b4a/2
  Subtract_5bf3e/1 -> Add_16486/1
  Constant_-1_2a73e/1 -> Product_aaf8d/1
  State_psi_q_SG_D_2_cf3b4/1 -> Add_16486/2
  Product_11a3c/1 -> Add_ebe0c/1
  Product_ac7a7/1 -> Add_11a5b/1
  Constant_-1_20001/1 -> Product_3a6bc/1
  Product_76501/1 -> Divide_227bb/1
  Constant_x_l_7fa88/1 -> Product_3a6bc/2
  Product_ca1c0/1 -> Add_da2e7/2
  Constant_x_qd_cb7b2/1 -> Subtract_835f9/1
  Add_c8b4a/1 -> Product_76501/1
  State_psi_gq_SG_D_2_de864/1 -> Product_9d612/1
  Add_ebe0c/1 -> Divide_be171/2
  Add_11a5b/1 -> Product_9d612/2
  Product_3a6bc/1 -> Add_50bbc/1
  Constant_x_qd_ec276/1 -> Add_50bbc/2
  State_psi_kq_SG_D_2_af7b7/1 -> Product_eb4cd/1
  Subtract_835f9/1 -> Product_eb4cd/2
  Divide_be171/1 -> Subtract_87c1c/2
  State_psi_kq_SG_D_2_65b80/1 -> Add_f5abf/2
  Product_eb4cd/1 -> Divide_be171/1
  Constant_x_qdd_16199/1 -> Divide_227bb/2
  Product_9d612/1 -> Divide_07110/1
  Add_50bbc/1 -> Divide_07110/2
  Constant_-1_68201/1 -> Product_f94e2/1
  Subtract_a81fe/1 -> Product_f94e2/2
  Add_f5abf/1 -> Subtract_dbe00/1
  Divide_227bb/1 -> Subtract_dbe00/2
  Product_aaf8d/1 -> Add_8589d/1
  Constant_x_qd_c6986/1 -> Add_8589d/2
  Divide_07110/1 -> Subtract_87c1c/1
  Product_f94e2/1 -> Product_16690/1
  Subtract_dbe00/1 -> Product_16690/2
  Add_8589d/1 -> Power_52a79/1
  Constant_2.0_6ec1a/1 -> Power_52a79/2
  Subtract_87c1c/1 -> Add_2a505/1
  State_psi_q_SG_D_2_77370/1 -> Add_2a505/2
  Product_16690/1 -> Divide_1429d/1
  Power_52a79/1 -> Divide_1429d/2
  Add_2a505/1 -> Divide_fcc0a/1
  Constant_x_qdd_9f9e6/1 -> Divide_fcc0a/2
  Constant_x_q_6c482/1 -> Subtract_82aca/1
  Divide_1429d/1 -> Subtract_aa209/1
  Divide_fcc0a/1 -> Subtract_aa209/2
  Divide_02b28/1 -> Blockout_d_psi_gq_SG_D_2_d0f45/1
  Constant_-1_5af4f/1 -> Product_e360d/1
  State_psi_gq_SG_D_2_6e475/1 -> Product_e360d/2
  Subtract_82aca/1 -> Product_ca1c0/1
  Subtract_aa209/1 -> Product_ca1c0/2
  Product_e360d/1 -> Add_da2e7/1
  Add_da2e7/1 -> Divide_02b28/1
  Constant_T_qd_6344d/1 -> Divide_02b28/2

== system case3/SG_D_2/d_psi_kq_SG_D_2_block ==
  note: d_psi_kq_SG_D_2 in case3
      | $-\frac{\psi _{\mathrm{gq},\mathrm{SG},D,2}+\psi _{\mathrm{kq},\mathrm{SG},D,2}+\frac{\left(x_{l}-x_{\mathrm{qd}}\right)\,\left(\psi _{q,\mathrm{SG},D,2}+\frac{\psi _{\mathrm{gq},\mathrm{SG},D,2}\,\left(x_{l}-x_{\mathrm{qdd}}\right)}{x_{l}-x_{\mathrm{qd}}}+\frac{\psi _{\mathrm{kq},\mathrm{SG},D,2}\,\left(x_{\mathrm{qd}}-x_{\mathrm{qdd}}\right)}{x_{l}-x_{\mathrm{qd}}}\right)}{x_{\mathrm{qdd}}}}{T_{\mathrm{qdd}}}$
      | Automatically generated on 2025-10-31 19:00:13 .
  State_psi_gq_SG_D_2_f7272 : Inport
  State_psi_kq_SG_D_2_8e84a : Inport  Port=2
  State_psi_gq_SG_D_2_fd868 : Inport  Port=3
  State_psi_kq_SG_D_2_a3af5 : Inport  Port=4
  State_psi_q_SG_D_2_baf03 : Inport  Port=5
  Add_00902 : Sum
  Add_b5ccb : Sum
  Add_ba2c1 : Sum
  Add_d5ef2 : Sum
  Add_ec228 : Sum
  Add_fbc59 : Sum
  Constant_-1_3a942 : Constant  Value=-1
  Constant_-1_9b3e4 : Constant  Value=-1
  Constant_-1_c3ecd : Constant  Value=-1
  Constant_-1_d4a84 : Constant  Value=-1
  Constant_-1_d717a : Constant  Value=-1
  Constant_T_qdd_f2ad8 : Constant  Value=T_qdd
  Constant_x_l_64757 : Constant  Value=x_l
  Constant_x_l_b298d : Constant  Value=x_l
  Constant_x_l_f7f1d : Constant  Value=x_l
  Constant_x_l_fee3a : Constant  Value=x_l
  Constant_x_qd_46692 : Constant  Value=x_qd
  Constant_x_qd_aff38 : Constant  Value=x_qd
  Constant_x_qd_b089f : Constant  Value=x_qd
  Constant_x_qd_f1c6e : Constant  Value=x_qd
  Constant_x_qdd_0095b : Constant  Value=x_qdd
  Constant_x_qdd_29715 : Constant  Value=x_qdd
  Constant_x_qdd_3653f : Constant  Value=x_qdd
  Divide_25819 : Product  Inputs=*/
  Divide_4350f : Product  Inputs=*/
  Divide_b1439 : Product  Inputs=*/
  Divide_f088a : Product  Inputs=*/
  Product_3180d : Product
  Product_37763 : Product
  Product_4a380 : Product
  Product_5ac7d : Product
  Product_85174 : Product
  Product_a1dad : Product
  Product_a8d15 : Product
  Product_c7c7b : Product
  Subtract_2ac74 : Sum  Inputs=+-
  Subtract_477d9 : Sum  Inputs=+-
  Subtract_54273 : Sum  Inputs=+-
  Blockout_d_psi_kq_SG_D_2_93807 : Outport
  wires:
  State_psi_kq_SG_D_2_8e84a/1 -> Subtract_477d9/2
  Constant_-1_d4a84/1 -> Product_c7c7b/1
  Constant_-1_d717a/1 -> Product_a1dad/1
  Constant_x_l_64757/1 -> Product_a1dad/2
  Constant_x_qdd_0095b/1 -> Add_00902/2
  Constant_x_l_f7f1d/1 -> Product_c7c7b/2
  Constant_x_qd_f1c6e/1 -> Subtract_2ac74/1
  Constant_T_qdd_f2ad8/1 -> Divide_4350f/2
  Constant_-1_c3ecd/1 -> Product_a8d15/1
  Product_a1dad/1 -> Add_00902/1
  Constant_x_qdd_29715/1 -> Subtract_2ac74/2
  Constant_x_l_b298d/1 -> Product_a8d15/2
  Divide_4350f/1 -> Blockout_d_psi_kq_SG_D_2_93807/1
  State_psi_gq_SG_D_2_fd868/1 -> Product_37763/1
  Add_00902/1 -> Product_37763/2
  Product_c7c7b/1 -> Add_ec228/1
  Constant_x_qd_aff38/1 -> Add_ec228/2
  Product_4a380/1 -> Divide_b1439/1
  State_psi_kq_SG_D_2_a3af5/1 -> Product_3180d/1
  Subtract_2ac74/1 -> Product_3180d/2
  Product_a8d15/1 -> Add_ba2c1/1
  Constant_x_qd_46692/1 -> Add_ba2c1/2
  Product_3180d/1 -> Divide_f088a/1
  Product_37763/1 -> Divide_25819/1
  Add_ec228/1 -> Divide_25819/2
  Add_ba2c1/1 -> Divide_f088a/2
  State_psi_q_SG_D_2_baf03/1 -> Add_fbc59/2
  Constant_-1_9b3e4/1 -> Product_85174/1
  Constant_x_l_fee3a/1 -> Product_85174/2
  Divide_25819/1 -> Subtract_54273/1
  Divide_f088a/1 -> Subtract_54273/2
  Product_85174/1 -> Add_b5ccb/1
  Constant_x_qd_b089f/1 -> Add_b5ccb/2
  Subtract_54273/1 -> Add_fbc59/1
  Constant_x_qdd_3653f/1 -> Divide_b1439/2
  Constant_-1_3a942/1 -> Product_5ac7d/1
  State_psi_gq_SG_D_2_f7272/1 -> Product_5ac7d/2
  Add_b5ccb/1 -> Product_4a380/1
  Add_fbc59/1 -> Product_4a380/2
  Product_5ac7d/1 -> Subtract_477d9/1
  Subtract_477d9/1 -> Add_d5ef2/1
  Divide_b1439/1 -> Add_d5ef2/2
  Add_d5ef2/1 -> Divide_4350f/1

== system case3/SG_D_2/d_psi_q_SG_D_2_block ==
  note: d_psi_q_SG_D_2 in case3
      | $2\,\pi \,f_{0}\,\left(v_{d,\mathrm{SG},D,2}\,\cos\left(\theta _{\mathrm{SG},D,2}\right)+v_{q,\mathrm{SG},D,2}\,\sin\left(\theta _{\mathrm{SG},D,2}\right)-\frac{R_{a}\,\left(\psi _{q,\mathrm{SG},D,2}+\frac{\psi _{\mathrm{gq},\mathrm{SG},D,2}\,\left(x_{l}-x_{\mathrm{qdd}}\right)}{x_{l}-x_{\mathrm{qd}}}+\frac{\psi _{\mathrm{kq},\mathrm{SG},D,2}\,\left(x_{\mathrm{qd}}-x_{\mathrm{qdd}}\right)}{x_{l}-x_{\mathrm{qd}}}\right)}{x_{\mathrm{qdd}}}-\frac{\psi _{d,\mathrm{SG},D,2}\,w_{\mathrm{SG},D,2}}{2\,f_{0}\,\pi }\right)$
      | Automatically generated on 2025-10-31 18:59:55 .
  State_psi_gq_SG_D_2_0e848 : Inport
  State_psi_kq_SG_D_2_c82e0 : Inport  Port=2
  State_psi_q_SG_D_2_7ccdb : Inport  Port=3
  Input_v_d_SG_D_2_cf2d7 : Inport  Port=4
  State_theta_SG_D_2_ef5e0 : Inport  Port=5
  Input_v_q_SG_D_2_6f15e : Inport  Port=6
  State_theta_SG_D_2_f1f7c : Inport  Port=7
  State_psi_d_SG_D_2_a8ebf : Inport  Port=8
  State_w_SG_D_2_01d6c : Inport  Port=9
  Add_450aa : Sum
  Add_4a2d6 : Sum
  Add_742a1 : Sum
  Add_b87d7 : Sum
  Add_ee110 : Sum
  Constant_-1_48a82 : Constant  Value=-1
  Constant_-1_4ae7c : Constant  Value=-1
  Constant_-1_8dd11 : Constant  Value=-1
  Constant_-2.0_d6bfc : Constant  Value=-2.0
  Constant_2.0_2ce82 : Constant  Value=2.0
  Constant_R_a_2a847 : Constant  Value=R_a
  Constant_f0_4a682 : Constant  Value=f0
  Constant_f0_7e0d8 : Constant  Value=f0
  Constant_pi_29ca8 : Constant  Value=pi
  Constant_pi_bfccd : Constant  Value=pi
  Constant_x_l_4542e : Constant  Value=x_l
  Constant_x_l_4656d : Constant  Value=x_l
  Constant_x_l_8c847 : Constant  Value=x_l
  Constant_x_qd_29c10 : Constant  Value=x_qd
  Constant_x_qd_c03fb : Constant  Value=x_qd
  Constant_x_qd_e0197 : Constant  Value=x_qd
  Constant_x_qdd_a4e62 : Constant  Value=x_qdd
  Constant_x_qdd_cf89b : Constant  Value=x_qdd
  Constant_x_qdd_e0945 : Constant  Value=x_qdd
  Divide_28cb1 : Product  Inputs=*/
  Divide_3bd99 : Product  Inputs=*/
  Divide_77f04 : Product  Inputs=*/
  Divide_b4b9c : Product  Inputs=*/
  MathFunc_cos_48a02 : Trigonometry  Operator=cos
  MathFunc_sin_d3a57 : Trigonometry
  Product_0e310 : Product
  Product_1070b : Product
  Product_2cb00 : Product
  Product_362e0 : Product
  Product_4bae3 : Product
  Product_4bf10 : Product
  Product_5c2bc : Product
  Product_66cd9 : Product
  Product_74246 : Product
  Product_75d7f : Product
  Product_9fd98 : Product
  Product_cdcc0 : Product
  Product_deb5d : Product
  Product_fa8a9 : Product
  Subtract_07e67 : Sum  Inputs=+-
  Subtract_37ddf : Sum  Inputs=+-
  Subtract_47bec : Sum  Inputs=+-
  Subtract_80c9c : Sum  Inputs=+-
  Blockout_d_psi_q_SG_D_2_96569 : Outport
  wires:
  Constant_x_qdd_cf89b/1 -> Subtract_37ddf/2
  Constant_x_l_4656d/1 -> Product_0e310/2
  Constant_-1_4ae7c/1 -> Product_deb5d/1
  Constant_x_l_4542e/1 -> Product_deb5d/2
  Product_deb5d/1 -> Add_4a2d6/1
  Constant_pi_bfccd/1 -> Product_362e0/2
  State_psi_gq_SG_D_2_0e848/1 -> Product_74246/1
  Constant_x_l_8c847/1 -> Product_2cb00/2
  State_w_SG_D_2_01d6c/1 -> Product_5c2bc/2
  Constant_x_qd_29c10/1 -> Add_ee110/2
  Constant_x_qdd_a4e62/1 -> Add_4a2d6/2
  Constant_2.0_2ce82/1 -> Product_362e0/1
  Constant_-1_8dd11/1 -> Product_2cb00/1
  Constant_x_qd_e0197/1 -> Subtract_37ddf/1
  Constant_-1_48a82/1 -> Product_0e310/1
  State_psi_q_SG_D_2_7ccdb/1 -> Add_450aa/2
  Add_4a2d6/1 -> Product_74246/2
  Product_362e0/1 -> Product_66cd9/1
  Product_2cb00/1 -> Add_b87d7/1
  Constant_pi_29ca8/1 -> Product_4bf10/2
  Constant_f0_7e0d8/1 -> Product_66cd9/2
  Constant_x_qd_c03fb/1 -> Add_b87d7/2
  State_psi_kq_SG_D_2_c82e0/1 -> Product_cdcc0/1
  Subtract_37ddf/1 -> Product_cdcc0/2
  Product_0e310/1 -> Add_ee110/1
  Input_v_q_SG_D_2_6f15e/1 -> Product_fa8a9/1
  Product_74246/1 -> Divide_3bd99/1
  Product_66cd9/1 -> Divide_b4b9c/2
  Add_b87d7/1 -> Divide_3bd99/2
  Product_cdcc0/1 -> Divide_77f04/1
  Add_ee110/1 -> Divide_77f04/2
  Divide_3bd99/1 -> Subtract_80c9c/1
  State_theta_SG_D_2_ef5e0/1 -> MathFunc_cos_48a02/1
  Divide_77f04/1 -> Subtract_80c9c/2
  Subtract_80c9c/1 -> Add_450aa/1
  MathFunc_cos_48a02/1 -> Product_1070b/2
  Constant_R_a_2a847/1 -> Product_4bae3/1
  Add_450aa/1 -> Product_4bae3/2
  State_theta_SG_D_2_f1f7c/1 -> MathFunc_sin_d3a57/1
  Product_4bae3/1 -> Divide_28cb1/1
  Product_4bf10/1 -> Product_75d7f/1
  Product_fa8a9/1 -> Subtract_47bec/2
  Constant_x_qdd_e0945/1 -> Divide_28cb1/2
  Input_v_d_SG_D_2_cf2d7/1 -> Product_1070b/1
  Add_742a1/1 -> Product_9fd98/2
  Divide_28cb1/1 -> Subtract_07e67/1
  Product_1070b/1 -> Subtract_07e67/2
  MathFunc_sin_d3a57/1 -> Product_fa8a9/2
  Product_9fd98/1 -> Blockout_d_psi_q_SG_D_2_96569/1
  State_psi_d_SG_D_2_a8ebf/1 -> Product_5c2bc/1
  Constant_-2.0_d6bfc/1 -> Product_4bf10/1
  Product_75d7f/1 -> Product_9fd98/1
  Subtract_07e67/1 -> Subtract_47bec/1
  Product_5c2bc/1 -> Divide_b4b9c/1
  Constant_f0_4a682/1 -> Product_75d7f/2
  Subtract_47bec/1 -> Add_742a1/1
  Divide_b4b9c/1 -> Add_742a1/2

== system case3/SG_D_2/d_theta_SG_D_2_block ==
  note: d_theta_SG_D_2 in case3
      | $w_{\mathrm{SG},D,2}-2\,\pi \,f_{0}$
      | Automatically generated on 2025-10-31 19:00:20 .
  State_w_SG_D_2_906f7 : Inport
  Add_4ed88 : Sum
  Constant_-2.0_31ae6 : Constant  Value=-2.0
  Constant_f0_83d23 : Constant  Value=f0
  Constant_pi_2f982 : Constant  Value=pi
  Product_351f3 : Product
  Product_4ba2f : Product
  Blockout_d_theta_SG_D_2_79f4e : Outport
  wires:
  Constant_-2.0_31ae6/1 -> Product_4ba2f/1
  Constant_pi_2f982/1 -> Product_4ba2f/2
  Add_4ed88/1 -> Blockout_d_theta_SG_D_2_79f4e/1
  Product_4ba2f/1 -> Product_351f3/1
  Constant_f0_83d23/1 -> Product_351f3/2
  Product_351f3/1 -> Add_4ed88/1
  State_w_SG_D_2_906f7/1 -> Add_4ed88/2
